simulink model "LC62_PIDControl_V6"  (R2022b)
settings: Solver=ode4  StartTime=0.0  StopTime=SimTime  FixedStep=1/500  RelTol=1e-3
model workspace (MAT data in the model file):
  Tr = 0.1
  freq = 0.002
  hover_w = 0.55
values from neighbouring files (symbols this model uses):
  b = 1.1    [initfun.m]
  c = 0.551    [initfun.m]
  Cll_beta = -0.0518    [initfun.m]
  Cll_del_A = -0.0369 * 5    (= -0.1845)    [initfun.m]
  Cll_del_R = 0.0026    [initfun.m]
  Cll_p = -0.4624    [initfun.m]
  Cll_r = 0.0218    [initfun.m]
  Cm_del_A = 0.001156    [initfun.m]
  Cm_del_E = -0.676    [initfun.m]
  Cn_beta = 0.0866    [initfun.m]
  Cn_del_A = -0.000385    [initfun.m]
  Cn_del_R = -0.0190    (= -0.019)    [initfun.m]
  Cn_p = -0.0048    [initfun.m]
  Cn_r = -0.0723    [initfun.m]
  Cy_beta = -1.1269    [initfun.m]
  Cy_del_R = 0.0534    [initfun.m]
  Cy_p = 0.0    (= 0)    [initfun.m]
  Cy_r = 0.2374    [initfun.m]
  d = 0.849    [initfun.m]
  dx1 = 0.9325+0.049    (= 0.9815)    [initfun.m]
  dx2 = 0.0725-0.049    (= 0.0235)    [initfun.m]
  dx3 = 1.1725-0.049    (= 1.1235)    [initfun.m]
  dy1 = 0.717 + temp_y    (= 0.717)    [initfun.m]
  dy2 = 0.717 - temp_y    (= 0.717)    [initfun.m]
  g = 9.81    [initfun.m]
  m = 41.97    [initfun.m]
  S = S1 + S2    (= 0.8522)    [initfun.m]
  S2 = 0.5898    [initfun.m]
undefined symbols (not defined in the file or in its folder): d2r, Earth, F, Light, MIL, sigbuilder_block, WGS84
libraries: simulink_extras x50, slpidlib x14, simulink x11, dspstat3 x5, aerolibwind2 x3, sharedTrackingLibrary x2, aerolibasang x2, aerolibtransform2 x2, robotcorelib x1, uavutilslib x1, uavalgslib x1, aerolibnav x1
(part 4 of 4)

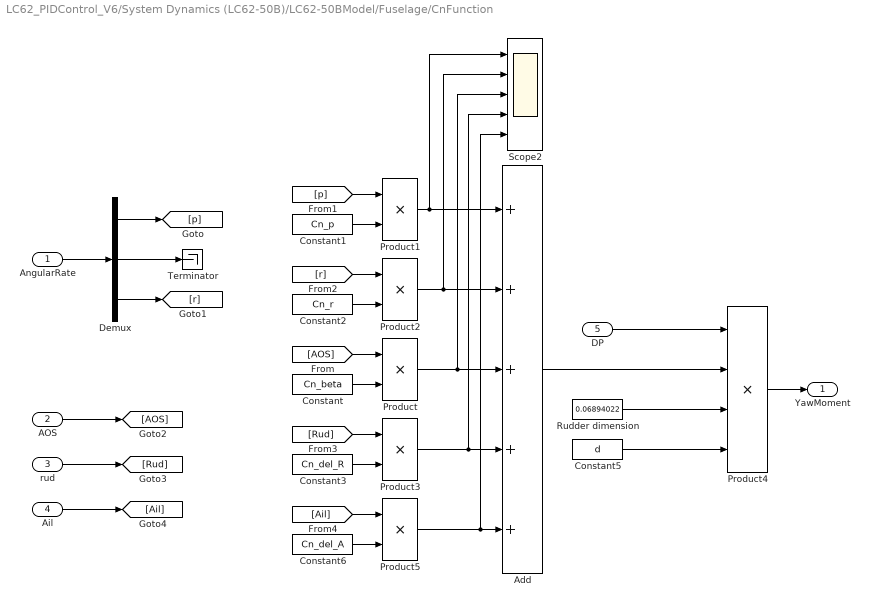
== system LC62_PIDControl_V6/System Dynamics (LC62-50B)/LC62-50BModel/Fuselage/CnFunction ==
  AngularRate : Inport
  AOS : Inport  Port=2
  rud : Inport  Port=3
  Ail : Inport  Port=4
  DP : Inport  Port=5
  Add : Sum  Inputs=+++++
  Constant : Constant  Value=Cn_beta
  Constant1 : Constant  Value=Cn_p
  Constant2 : Constant  Value=Cn_r
  Constant3 : Constant  Value=Cn_del_R
  Constant5 : Constant  Value=d
  Constant6 : Constant  Value=Cn_del_A
  Demux : Demux  Outputs=3
  Product{,1..3,5} (5 alike) : Product
  Product4 : Product  Inputs=4
  Rudder dimension : Constant  Value=0.06894022
  Scope2 : Scope  NumInputPorts=5
  Terminator : Terminator
  YawMoment : Outport
  wires:
  Product4/1 -> YawMoment/1
  Constant5/1 -> Product4/4
  Product2/1 -> Scope2/2, Add/2
  Product3/1 -> Scope2/4, Add/4
  Constant3/1 -> Product3/2
  [Rud] -> Product3/1
  Constant2/1 -> Product2/2
  [r] -> Product2/1
  [p] -> Product1/1
  Constant1/1 -> Product1/2
  Constant/1 -> Product/2
  [AOS] -> Product/1
  rud/1 -> [Rud]
  AOS/1 -> [AOS]
  Demux/2 -> Terminator/1
  Demux/3 -> [r]
  Demux/1 -> [p]
  AngularRate/1 -> Demux/1
  Rudder dimension/1 -> Product4/3
  Add/1 -> Product4/2
  Product1/1 -> Scope2/1, Add/1
  Product/1 -> Scope2/3, Add/3
  Ail/1 -> [Ail]
  DP/1 -> Product4/1
  [Ail] -> Product5/1
  Constant6/1 -> Product5/2
  Product5/1 -> Scope2/5, Add/5

== system LC62_PIDControl_V6/System Dynamics (LC62-50B)/LC62-50BModel/Fuselage/CyFunction ==
  AngularRate : Inport
  AOS : Inport  Port=2
  Rud : Inport  Port=3
  DP : Inport  Port=4
  Add : Sum  Inputs=++++
  Constant : Constant  Value=Cy_beta
  Constant1 : Constant  Value=Cy_p
  Constant2 : Constant  Value=Cy_r
  Constant4 : Constant  Value=S
  Constant6 : Constant  Value=Cy_del_R
  Demux : Demux  Outputs=3
  Product{,1..2,5} (4 alike) : Product
  Product4 : Product  Inputs=3
  Terminator : Terminator
  y force : Outport
  wires:
  DP/1 -> Product4/1
  Rud/1 -> [Rud]
  [Rud] -> Product5/1
  Constant6/1 -> Product5/2
  Product4/1 -> y force/1
  Constant4/1 -> Product4/3
  Add/1 -> Product4/2
  Constant2/1 -> Product2/2
  [r] -> Product2/1
  [p] -> Product1/1
  Constant1/1 -> Product1/2
  Constant/1 -> Product/2
  [AOS] -> Product/1
  AOS/1 -> [AOS]
  Demux/2 -> Terminator/1
  Demux/3 -> [r]
  Demux/1 -> [p]
  AngularRate/1 -> Demux/1
  Product5/1 -> Add/4
  Product/1 -> Add/3
  Product2/1 -> Add/2
  Product1/1 -> Add/1

== system LC62_PIDControl_V6/System Dynamics (LC62-50B)/LC62-50BModel/Pusher/Rotor01 ==
  In1 : Inport
  1-D Lookup Table : Lookup_n-D  NumberOfTableDimensions=1  BreakpointsForDimension1=[1000,1200,1255,1310,1365,1420,1475,1530,1585,1640,1695,1750]  Table=[0,1.39,4.22,7.89,12.36,17.60,23.19,29.99,39.09,46.14,52.67,59.69]  ExtrapMethod=Clip  UseLastTableValue=on  InternalRulePriority=Speed  RndMeth=Simplest
  1-D Lookup Table1 : Lookup_n-D  NumberOfTableDimensions=1  BreakpointsForDimension1=[1000,1200,1255,1310,1365,1420,1475,1530,1585,1640,1695,1750]  Table=[0,0.12,0.35,0.66,1.04,1.47,1.93,2.50,3.25,3.83,4.35,4.95]  ExtrapMethod=Clip  UseLastTableValue=on  InternalRulePriority=Speed  RndMeth=Simplest
  Thrust : Outport
  Torque : Outport  Port=2
  wires:
  1-D Lookup Table/1 -> Thrust/1
  In1/1 -> 1-D Lookup Table1/1, 1-D Lookup Table/1
  1-D Lookup Table1/1 -> Torque/1

== system LC62_PIDControl_V6/System Dynamics (LC62-50B)/LC62-50BModel/Pusher/Rotor02 ==
  In1 : Inport
  1-D Lookup Table : Lookup_n-D  NumberOfTableDimensions=1  BreakpointsForDimension1=[1000,1200,1255,1310,1365,1420,1475,1530,1585,1640,1695,1750]  Table=[0,1.39,4.22,7.89,12.36,17.60,23.19,29.99,39.09,46.14,52.67,59.69]  ExtrapMethod=Clip  UseLastTableValue=on  InternalRulePriority=Speed  RndMeth=Simplest
  1-D Lookup Table1 : Lookup_n-D  NumberOfTableDimensions=1  BreakpointsForDimension1=[1000,1200,1255,1310,1365,1420,1475,1530,1585,1640,1695,1750]  Table=[0,0.12,0.35,0.66,1.04,1.47,1.93,2.50,3.25,3.83,4.35,4.95]  ExtrapMethod=Clip  UseLastTableValue=on  InternalRulePriority=Speed  RndMeth=Simplest
  Thrust : Outport
  Torque : Outport  Port=2
  wires:
  1-D Lookup Table1/1 -> Torque/1
  In1/1 -> 1-D Lookup Table/1, 1-D Lookup Table1/1
  1-D Lookup Table/1 -> Thrust/1

== system LC62_PIDControl_V6/System Dynamics (LC62-50B)/LC62-50BModel/VTOLRotor/Compansation ==
  In1 : Inport
  Constant4 : Constant  Value=0.5
  Gain : Gain  Gain=2
  Gain2 : Gain
  Product : Product
  Radians to Degrees : simulink_extras/Transformations/Radians to Degrees
  Radians to Degrees1 : simulink_extras/Transformations/Radians to Degrees
  Radians to Degrees2 : simulink_extras/Transformations/Radians to Degrees
  Selector : Selector  InputPortWidth=3  IndexOptions=Index vector (dialog)  Indices=2  OutputSizes=1
  Selector1 : Selector  InputPortWidth=3  IndexOptions=Index vector (dialog)  Indices=1  OutputSizes=1
  Selector2 : Selector  InputPortWidth=3  IndexOptions=Index vector (dialog)  Indices=3  OutputSizes=1
  rolling : Outport
  Pitching : Outport  Port=2
  Yawing : Outport  Port=3
  wires:
  In1/1 -> Selector2/1, Selector1/1, Selector/1
  Selector/1 -> Radians to Degrees/1
  Radians to Degrees/1 -> Gain/1
  Selector1/1 -> Radians to Degrees1/1
  Selector2/1 -> Radians to Degrees2/1
  Radians to Degrees2/1 -> Gain2/1
  Radians to Degrees1/1 -> [p]
  [p] -> Product/1
  Constant4/1 -> Product/2
  Product/1 -> rolling/1
  Gain/1 -> Pitching/1
  Gain2/1 -> Yawing/1

== system LC62_PIDControl_V6/System Dynamics (LC62-50B)/LC62-50BModel/VTOLRotor/Rotor01 ==
  note: Torque Equation : y = -6.3961x^3+12.092x^2-0.3156x
  note: Thrust Equation : y = -19281x^3+36503x^2-992.75x
  note: PWM2Command(1000~2000 -> 0 ~ 1)
  In1 : Inport
  Add : Sum  Inputs=-+-
  Add1 : Sum  Inputs=-+-
  Constant : Constant  Value=1000
  Constant1 : Constant  Value=3
  Constant2 : Constant  Value=2
  Constant3 : Constant  Value=3
  Constant4 : Constant  Value=2
  Gain : Gain  Gain=1/1000
  Gain1 : Gain  Gain=19281
  Gain2 : Gain  Gain=36503
  Gain3 : Gain  Gain=992.75
  Gain4 : Gain  Gain=6.3961
  Gain5 : Gain  Gain=12.092
  Gain6 : Gain  Gain=0.3156
  Gain7 : Gain  Gain=9.81/1000
  Math Function{,1..3} (4 alike) : Math  Operator=pow
  Saturation : Saturate  UpperLimit=1  LowerLimit=0
  Sum : Sum  Inputs=|+-
  Thrust : Outport
  Torque : Outport  Port=2
  tag scope: PWM1_out=global
  wires:
  In1/1 -> Sum/1
  Constant/1 -> Sum/2
  Sum/1 -> Gain/1
  Constant1/1 -> Math Function/2
  Math Function/1 -> Gain1/1
  Gain1/1 -> Add/1
  Gain2/1 -> Add/2
  Math Function1/1 -> Gain2/1
  Constant2/1 -> Math Function1/2
  Gain3/1 -> Add/3
  Add/1 -> Gain7/1
  Gain5/1 -> Add1/2
  Add1/1 -> Torque/1
  Math Function2/1 -> Gain4/1
  Gain/1 -> [PWM1_out], Saturation/1
  Constant4/1 -> Math Function3/2
  Math Function3/1 -> Gain5/1
  Gain4/1 -> Add1/1
  Gain6/1 -> Add1/3
  Constant3/1 -> Math Function2/2
  Gain7/1 -> Thrust/1
  Saturation/1 -> Gain6/1, Math Function3/1, Math Function2/1, Gain3/1, Math Function1/1, Math Function/1

== system LC62_PIDControl_V6/System Dynamics (LC62-50B)/LC62-50BModel/VTOLRotor/Rotor02 ==
  note: Torque Equation : y = -6.3961x^3+12.092x^2-0.3156x
  note: Thrust Equation : y = -19281x^3+36503x^2-992.75x
  note: PWM2Command(1000~2000 -> 0 ~ 1)
  In1 : Inport
  Add : Sum  Inputs=-+-
  Add1 : Sum  Inputs=-+-
  Constant : Constant  Value=1000
  Constant1 : Constant  Value=3
  Constant2 : Constant  Value=2
  Constant3 : Constant  Value=3
  Constant4 : Constant  Value=2
  Gain : Gain  Gain=1/1000
  Gain1 : Gain  Gain=19281
  Gain2 : Gain  Gain=36503
  Gain3 : Gain  Gain=992.75
  Gain4 : Gain  Gain=6.3961
  Gain5 : Gain  Gain=12.092
  Gain6 : Gain  Gain=0.3156
  Gain7 : Gain  Gain=9.81/1000
  Math Function{,1..3} (4 alike) : Math  Operator=pow
  Saturation : Saturate  UpperLimit=1  LowerLimit=0
  Sum : Sum  Inputs=|+-
  Thrust : Outport
  Torque : Outport  Port=2
  tag scope: PWM2_out=global
  wires:
  In1/1 -> Sum/1
  Constant/1 -> Sum/2
  Sum/1 -> Gain/1
  Constant1/1 -> Math Function/2
  Math Function/1 -> Gain1/1
  Gain1/1 -> Add/1
  Gain2/1 -> Add/2
  Math Function1/1 -> Gain2/1
  Constant2/1 -> Math Function1/2
  Gain3/1 -> Add/3
  Add/1 -> Gain7/1
  Gain5/1 -> Add1/2
  Add1/1 -> Torque/1
  Math Function2/1 -> Gain4/1
  Gain/1 -> [PWM2_out], Saturation/1
  Constant4/1 -> Math Function3/2
  Math Function3/1 -> Gain5/1
  Gain4/1 -> Add1/1
  Gain6/1 -> Add1/3
  Constant3/1 -> Math Function2/2
  Gain7/1 -> Thrust/1
  Saturation/1 -> Gain6/1, Math Function3/1, Math Function2/1, Gain3/1, Math Function1/1, Math Function/1

== system LC62_PIDControl_V6/System Dynamics (LC62-50B)/LC62-50BModel/VTOLRotor/Rotor03 ==
  note: Torque Equation : y = -6.3961x^3+12.092x^2-0.3156x
  note: Thrust Equation : y = -19281x^3+36503x^2-992.75x
  note: PWM2Command(1000~2000 -> 0 ~ 1)
  In1 : Inport
  Add : Sum  Inputs=-+-
  Add1 : Sum  Inputs=-+-
  Constant : Constant  Value=1000
  Constant1 : Constant  Value=3
  Constant2 : Constant  Value=2
  Constant3 : Constant  Value=3
  Constant4 : Constant  Value=2
  Gain : Gain  Gain=1/1000
  Gain1 : Gain  Gain=19281
  Gain2 : Gain  Gain=36503
  Gain3 : Gain  Gain=992.75
  Gain4 : Gain  Gain=6.3961
  Gain5 : Gain  Gain=12.092
  Gain6 : Gain  Gain=0.3156
  Gain7 : Gain  Gain=9.81/1000
  Math Function{,1..3} (4 alike) : Math  Operator=pow
  Saturation : Saturate  UpperLimit=1  LowerLimit=0
  Sum : Sum  Inputs=|+-
  Thrust : Outport
  Torque : Outport  Port=2
  tag scope: PWM3_out=global
  wires:
  In1/1 -> Sum/1
  Constant/1 -> Sum/2
  Sum/1 -> Gain/1
  Constant1/1 -> Math Function/2
  Math Function/1 -> Gain1/1
  Gain1/1 -> Add/1
  Gain2/1 -> Add/2
  Math Function1/1 -> Gain2/1
  Constant2/1 -> Math Function1/2
  Gain3/1 -> Add/3
  Add/1 -> Gain7/1
  Gain5/1 -> Add1/2
  Add1/1 -> Torque/1
  Math Function2/1 -> Gain4/1
  Gain/1 -> [PWM3_out], Saturation/1
  Constant4/1 -> Math Function3/2
  Math Function3/1 -> Gain5/1
  Gain4/1 -> Add1/1
  Gain6/1 -> Add1/3
  Constant3/1 -> Math Function2/2
  Gain7/1 -> Thrust/1
  Saturation/1 -> Gain6/1, Math Function3/1, Math Function2/1, Gain3/1, Math Function1/1, Math Function/1

== system LC62_PIDControl_V6/System Dynamics (LC62-50B)/LC62-50BModel/VTOLRotor/Rotor04 ==
  note: Torque Equation : y = -6.3961x^3+12.092x^2-0.3156x
  note: Thrust Equation : y = -19281x^3+36503x^2-992.75x
  note: PWM2Command(1000~2000 -> 0 ~ 1)
  In1 : Inport
  Add : Sum  Inputs=-+-
  Add1 : Sum  Inputs=-+-
  Constant : Constant  Value=1000
  Constant1 : Constant  Value=3
  Constant2 : Constant  Value=2
  Constant3 : Constant  Value=3
  Constant4 : Constant  Value=2
  Gain : Gain  Gain=1/1000
  Gain1 : Gain  Gain=19281
  Gain2 : Gain  Gain=36503
  Gain3 : Gain  Gain=992.75
  Gain4 : Gain  Gain=6.3961
  Gain5 : Gain  Gain=12.092
  Gain6 : Gain  Gain=0.3156
  Gain7 : Gain  Gain=9.81/1000
  Math Function{,1..3} (4 alike) : Math  Operator=pow
  Saturation : Saturate  UpperLimit=1  LowerLimit=0
  Sum : Sum  Inputs=|+-
  Thrust : Outport
  Torque : Outport  Port=2
  tag scope: PWM4_out=global
  wires:
  In1/1 -> Sum/1
  Constant/1 -> Sum/2
  Sum/1 -> Gain/1
  Constant1/1 -> Math Function/2
  Math Function/1 -> Gain1/1
  Gain1/1 -> Add/1
  Gain2/1 -> Add/2
  Math Function1/1 -> Gain2/1
  Constant2/1 -> Math Function1/2
  Gain3/1 -> Add/3
  Add/1 -> Gain7/1
  Gain5/1 -> Add1/2
  Add1/1 -> Torque/1
  Math Function2/1 -> Gain4/1
  Gain/1 -> [PWM4_out], Saturation/1
  Constant4/1 -> Math Function3/2
  Math Function3/1 -> Gain5/1
  Gain4/1 -> Add1/1
  Gain6/1 -> Add1/3
  Constant3/1 -> Math Function2/2
  Gain7/1 -> Thrust/1
  Saturation/1 -> Gain6/1, Math Function3/1, Math Function2/1, Gain3/1, Math Function1/1, Math Function/1

== system LC62_PIDControl_V6/System Dynamics (LC62-50B)/LC62-50BModel/VTOLRotor/Rotor05 ==
  note: Torque Equation : y = -6.3961x^3+12.092x^2-0.3156x
  note: Thrust Equation : y = -19281x^3+36503x^2-992.75x
  note: PWM2Command(1000~2000 -> 0 ~ 1)
  In1 : Inport
  Add : Sum  Inputs=-+-
  Add1 : Sum  Inputs=-+-
  Constant : Constant  Value=1000
  Constant1 : Constant  Value=3
  Constant2 : Constant  Value=2
  Constant3 : Constant  Value=3
  Constant4 : Constant  Value=2
  Gain : Gain  Gain=1/1000
  Gain1 : Gain  Gain=19281
  Gain2 : Gain  Gain=36503
  Gain3 : Gain  Gain=992.75
  Gain4 : Gain  Gain=6.3961
  Gain5 : Gain  Gain=12.092
  Gain6 : Gain  Gain=0.3156
  Gain7 : Gain  Gain=9.81/1000
  Math Function{,1..3} (4 alike) : Math  Operator=pow
  Saturation : Saturate  UpperLimit=1  LowerLimit=0
  Sum : Sum  Inputs=|+-
  Thrust : Outport
  Torque : Outport  Port=2
  tag scope: PWM5_out=global
  wires:
  In1/1 -> Sum/1
  Constant/1 -> Sum/2
  Sum/1 -> Gain/1
  Constant1/1 -> Math Function/2
  Math Function/1 -> Gain1/1
  Gain1/1 -> Add/1
  Gain2/1 -> Add/2
  Math Function1/1 -> Gain2/1
  Constant2/1 -> Math Function1/2
  Gain3/1 -> Add/3
  Add/1 -> Gain7/1
  Gain5/1 -> Add1/2
  Add1/1 -> Torque/1
  Math Function2/1 -> Gain4/1
  Gain/1 -> [PWM5_out], Saturation/1
  Constant4/1 -> Math Function3/2
  Math Function3/1 -> Gain5/1
  Gain4/1 -> Add1/1
  Gain6/1 -> Add1/3
  Constant3/1 -> Math Function2/2
  Gain7/1 -> Thrust/1
  Saturation/1 -> Gain6/1, Math Function3/1, Math Function2/1, Gain3/1, Math Function1/1, Math Function/1

== system LC62_PIDControl_V6/System Dynamics (LC62-50B)/LC62-50BModel/VTOLRotor/Rotor06 ==
  note: Torque Equation : y = -6.3961x^3+12.092x^2-0.3156x
  note: Thrust Equation : y = -19281x^3+36503x^2-992.75x
  note: PWM2Command(1000~2000 -> 0 ~ 1)
  In1 : Inport
  Add : Sum  Inputs=-+-
  Add1 : Sum  Inputs=-+-
  Constant : Constant  Value=1000
  Constant1 : Constant  Value=3
  Constant2 : Constant  Value=2
  Constant3 : Constant  Value=3
  Constant4 : Constant  Value=2
  Gain : Gain  Gain=1/1000
  Gain1 : Gain  Gain=19281
  Gain2 : Gain  Gain=36503
  Gain3 : Gain  Gain=992.75
  Gain4 : Gain  Gain=6.3961
  Gain5 : Gain  Gain=12.092
  Gain6 : Gain  Gain=0.3156
  Gain7 : Gain  Gain=9.81/1000
  Math Function{,1..3} (4 alike) : Math  Operator=pow
  Saturation : Saturate  UpperLimit=1  LowerLimit=0
  Sum : Sum  Inputs=|+-
  Thrust : Outport
  Torque : Outport  Port=2
  tag scope: PWM6_out=global
  wires:
  In1/1 -> Sum/1
  Constant/1 -> Sum/2
  Sum/1 -> Gain/1
  Constant1/1 -> Math Function/2
  Math Function/1 -> Gain1/1
  Gain1/1 -> Add/1
  Gain2/1 -> Add/2
  Math Function1/1 -> Gain2/1
  Constant2/1 -> Math Function1/2
  Gain3/1 -> Add/3
  Add/1 -> Gain7/1
  Gain5/1 -> Add1/2
  Add1/1 -> Torque/1
  Math Function2/1 -> Gain4/1
  Gain/1 -> [PWM6_out], Saturation/1
  Constant4/1 -> Math Function3/2
  Math Function3/1 -> Gain5/1
  Gain4/1 -> Add1/1
  Gain6/1 -> Add1/3
  Constant3/1 -> Math Function2/2
  Gain7/1 -> Thrust/1
  Saturation/1 -> Gain6/1, Math Function3/1, Math Function2/1, Gain3/1, Math Function1/1, Math Function/1

== system LC62_PIDControl_V6/System Dynamics (LC62-50B)/LC62-50BModel/VTOLRotor/Subsystem ==
  note: R1 : mid right
      | R2 : mid left
      | R3 : front left
      | R4 : rear right
      | R5 : front right
      | R6 : rear left
  Thrust 1 : Inport
  Thrust 2 : Inport  Port=2
  Thrust 3 : Inport  Port=3
  Thrust 4 : Inport  Port=4
  Thrust 5 : Inport  Port=5
  Thrust 6 : Inport  Port=6
  Add1 : Sum
  Add2 : Sum  Inputs=+++
  Add3 : Sum  Inputs=+-
  Add4 : Sum  Inputs=+++
  Add5 : Sum
  Add6 : Sum
  Add7 : Sum  Inputs=+--
  Constant : Constant  Value=1.0525
  Constant1 : Constant  Value=dy1
  Constant2 : Constant  Value=dy2
  Constant3 : Constant  Value=dx1
  Constant4 : Constant  Value=dx2
  Constant5 : Constant  Value=dx3
  Constant6 : Constant  Value=0
  Constant7 : Constant  Value=1.0525
  Manual Switch : ManualSwitch
  Manual Switch1 : ManualSwitch
  Manual Switch2 : ManualSwitch
  Product{,1..4} (5 alike) : Product
  RollingMoment : Outport
  PitchmingMoment : Outport  Port=2
  wires:
  Add2/1 -> Product/2
  Product1/1 -> Add3/2  "dy2(F1+F4+F5)"
  Add4/1 -> Product1/2
  Constant1/1 -> Product/1
  Product/1 -> Add3/1  "dy1(F2+F3+F6)"
  Constant2/1 -> Product1/1
  Add1/1 -> Product2/2
  Add5/1 -> Product3/2
  Add6/1 -> Product4/2
  Product2/1 -> Add7/1  "dx1(F3+F5)"
  Product3/1 -> Add7/2  "dx2(F1+F2)"
  Product4/1 -> Add7/3  "dx3(F4+F6)"
  Thrust 3/1 -> Add1/1, Add2/1
  Thrust 2/1 -> Add5/1, Add2/2
  Thrust 6/1 -> Add6/1, Add2/3
  Thrust 5/1 -> Add1/2, Add4/1
  Thrust 1/1 -> Add5/2, Add4/2
  Thrust 4/1 -> Add6/2, Add4/3
  Add7/1 -> PitchmingMoment/1
  Add3/1 -> RollingMoment/1
  Constant/1 -> Manual Switch/2
  Manual Switch/1 -> Product2/1
  Constant3/1 -> Manual Switch/1
  Manual Switch1/1 -> Product3/1
  Constant4/1 -> Manual Switch1/1
  Constant6/1 -> Manual Switch1/2
  Manual Switch2/1 -> Product4/1
  Constant5/1 -> Manual Switch2/1
  Constant7/1 -> Manual Switch2/2

== matlab function LC62_PIDControl_V6/Fault detection module/Residual 1 (r1)/az_pwm ==
  data: PWM input; az_pwm output
function az_pwm = fcn(PWM)
m = 41.97;              % kg

% Thrust-PWM relationship
K = 9.81/1000;                                                  % 단위([g] -> [N])와 PWM 0~1 사이로 정규화하기위해 곱해진 텀
a = -19281; b = 36503; c = -992.75;               % 추력 테스트 결과 방정식의 계수

T1 = K*(a*PWM(1)^3 + b*PWM(1)^2 + c*PWM(1));
T2 = K*(a*PWM(2)^3 + b*PWM(2)^2 + c*PWM(2));
T3 = K*(a*PWM(3)^3 + b*PWM(3)^2 + c*PWM(3));
T4 = K*(a*PWM(4)^3 + b*PWM(4)^2 + c*PWM(4));
T5 = K*(a*PWM(5)^3 + b*PWM(5)^2 + c*PWM(5));
T6 = K*(a*PWM(6)^3 + b*PWM(6)^2 + c*PWM(6));

az_pwm = (T1 + T2 + T3 + T4 + T5 + T6)/m;

== matlab function LC62_PIDControl_V6/Sensor and Fault injection/IMU sensor (MPU-6000)/Rotation MTX : Rbi (inertial to body) ==
  data: EulerAngle input; Rbi output
function Rbi = fcn(EulerAngle)
phi   = EulerAngle(1);
theta = EulerAngle(2);
psi   = EulerAngle(3);

Rib = [cos(theta)*cos(psi) sin(phi)*sin(theta)*cos(psi)-cos(phi)*sin(psi) cos(phi)*sin(theta)*cos(psi)+sin(phi)*sin(psi);
       cos(theta)*sin(psi) sin(phi)*sin(theta)*sin(psi)+cos(phi)*cos(psi) cos(phi)*sin(theta)*sin(psi)-sin(phi)*cos(psi);
       -sin(theta)         sin(phi)*cos(theta)                            cos(phi)*cos(theta)];
Rbi = Rib';
% Rib = body to inertial frame rotational matrix
% Rbi = inertial to body frame rotational matrix

== matlab function LC62_PIDControl_V6/PID Controller/Control Allocation (Control Mixer) ==
  data: u_phi input; mc1 output; u_theta input; u_psi input; u_z input; mc2 output; mc3 output; mc4 output; mc5 output; mc6 output
function [mc1, mc2, mc3, mc4, mc5, mc6] = fcn(u_phi, u_theta, u_psi, u_z)
% 1번, 2번 모터 중심과 무게중심이 동일 선상에 있다고 가정(Assume "dx2=0")
u = [u_z; u_phi; u_theta; u_psi];
A = [
    1 -1  0 -1
    1  1  0  1
    1  1  1 -1
    1 -1 -1  1
    1 -1  1  1
    1  1 -1 -1
    ];
MC = A*u;

mc1 = MC(1); mc2 = MC(2); mc3 = MC(3); 
mc4 = MC(4); mc5 = MC(5); mc6 = MC(6);

== matlab function LC62_PIDControl_V6/Sensor and Fault injection/az_pwm ==
  data: PWM input; az_pwm output
function az_pwm = fcn(PWM)
m = 41.97;              % kg

% Thrust-PWM relationship
K = 9.81/1000;                                                  % 단위([g] -> [N])와 PWM 0~1 사이로 정규화하기위해 곱해진 텀
a = -19281; b = 36503; c = -992.75;               % 추력 테스트 결과 방정식의 계수

T1 = K*(a*PWM(1)^3 + b*PWM(1)^2 + c*PWM(1));
T2 = K*(a*PWM(2)^3 + b*PWM(2)^2 + c*PWM(2));
T3 = K*(a*PWM(3)^3 + b*PWM(3)^2 + c*PWM(3));
T4 = K*(a*PWM(4)^3 + b*PWM(4)^2 + c*PWM(4));
T5 = K*(a*PWM(5)^3 + b*PWM(5)^2 + c*PWM(5));
T6 = K*(a*PWM(6)^3 + b*PWM(6)^2 + c*PWM(6));

az_pwm = (T1 + T2 + T3 + T4 + T5 + T6)/m;

== matlab function LC62_PIDControl_V6/Fault detection module/az_pwm ==
  data: PWM input; az_pwm output
function az_pwm = fcn(PWM)
m = 41.97;              % kg

% Thrust-PWM relationship
K = 9.81/1000;                                                  % 단위([g] -> [N])와 PWM 0~1 사이로 정규화하기위해 곱해진 텀
a = -19281; b = 36503; c = -992.75;               % 추력 테스트 결과 방정식의 계수

T1 = K*(a*PWM(1)^3 + b*PWM(1)^2 + c*PWM(1));
T2 = K*(a*PWM(2)^3 + b*PWM(2)^2 + c*PWM(2));
T3 = K*(a*PWM(3)^3 + b*PWM(3)^2 + c*PWM(3));
T4 = K*(a*PWM(4)^3 + b*PWM(4)^2 + c*PWM(4));
T5 = K*(a*PWM(5)^3 + b*PWM(5)^2 + c*PWM(5));
T6 = K*(a*PWM(6)^3 + b*PWM(6)^2 + c*PWM(6));

az_pwm = (T1 + T2 + T3 + T4 + T5 + T6)/m;

== matlab function LC62_PIDControl_V6/Position and Acceleration Control/Acceleration Control/Multirotor Acceleration Control ==
  data: acc input; roll output; pitch output; yaw input
function [roll, pitch] = accControl(acc, yaw)

    xddot = acc(1);
    yddot = acc(2);
    zddot = acc(3);
    Gravity = 9.81;

    pitch = atan2((-xddot*cos(yaw)-yddot*sin(yaw)), ( -zddot + Gravity));
    roll = atan2(((-xddot*sin(yaw)+yddot*cos(yaw))*cos(pitch)), (-zddot+Gravity));
    
end

== matlab function LC62_PIDControl_V6/Fault detection module/EKF 2/MATLAB Function ==
  data: acc input; phi output; theta output
function [phi, theta] = fcn(acc)
ax = acc(1);
ay = acc(2);
az = acc(3);

phi = atan(ay./az);
theta = atan(ax./sqrt(ay.^2+az.^2));

== matlab function LC62_PIDControl_V6/Fault detection module/Residual 1 (r1)/MATLAB Function ==
  data: xEstimated input; u input; yhat output
function yhat = generatePredictedOutput(xEstimated,u)
%% xhat[k|k-1]
xPredicted = EKF1_fn_fx(xEstimated,u); 
%% y[k|k-1]
yhat = EKF1_fn_hx(xPredicted);
end

== matlab function LC62_PIDControl_V6/Fault detection module/Residual 2 (r2)/MATLAB Function ==
  data: xEstimated input; yhat output; rates input
function yhat = generatePredictedOutput(xEstimated,rates)
%% xhat[k|k-1]
xPredicted = EKF2_fn_fx(xEstimated,rates); 
%% y[k|k-1]
yhat = EKF2_fn_hx(xPredicted);
end

== matlab function LC62_PIDControl_V6/Fault detection module/FDI ==
  data: r1 input; y output; r2 input
function y = fcn(r1, r2)
lamb_p = 5e-4; % 8e-4; for Hexacopter
lamb_q = 5e-4;% 8e-4; for Hexacopter
lamb_r  = 5e-4;% 8e-4; for Hexacopter
% lamb_az = 1;    %0.96; for Hexacopter

lamb_phi = 1.4e-4; %11.5e-4; for Hexacopter
lamb_the = 1.4e-4; %11e-4; for Hexacopter

r_p = r1(1); r_q = r1(2); r_r = r1(3);
% r_az = r1(4);

r_phi = r2(1); r_the = r2(2);

y=1;
while y==1
    if r_p < lamb_p && r_q < lamb_q && r_r < lamb_r && r_phi < lamb_phi  && r_the < lamb_the
        y = 1;   % y = 1 : fault-free
    elseif r_p < lamb_p && r_q < lamb_q && r_r < lamb_r && r_phi >= lamb_phi && r_the >= lamb_the
        y = 2;   % y = 2 : Accelerometer fault
    elseif r_p >= lamb_p && r_q >= lamb_q && r_r >= lamb_r && r_phi >= lamb_phi && r_the >= lamb_the
        y = 3;   % y = 3 : Gyroscope fault
    % 가속도계 축별 고장진단
    elseif r_p < lamb_p && r_q < lamb_q && r_r < lamb_r && r_phi < lamb_phi && r_the >= lamb_the
        y = 21;  % y = 21: a_x 고장
    elseif r_p < lamb_p && r_q < lamb_q && r_r < lamb_r && r_phi >= lamb_phi && r_the < lamb_the
        y = 22;  % y = 22: a_y 고장
    % 자이로스코프 축별 고장진단
    elseif r_p >= lamb_p && r_q < lamb_q && r_r < lamb_r && r_phi >= lamb_phi && r_the < lamb_the
        y = 31;  % y = 31: p 고장
    elseif r_p < lamb_p && r_q >= lamb_q && r_r < lamb_r && r_phi < lamb_phi && r_the >= lamb_the
        y = 32;  % y = 32: q 고장
    elseif r_p >= lamb_p && r_q < lamb_q && r_r >= lamb_r && r_phi >= lamb_phi && r_the < lamb_the
        y = 33;  % y = 33: r 고장
    end
    break
end
